simulink model "tinydl"  (R2025b)
settings: Solver=FixedStepAuto  StartTime=0.0  StopTime=inf  RelTol=1e-3  EnableMultiTasking=on
libraries: arduinolib x8
settings Model: ExtModeTrigDuration=2  Creator=Dogukan.kilinc  LastModifiedBy=Dogukan.kilinc
settings SolverCC: AutoInsertRateTranBlk=on
settings DataIOCC: ReturnWorkspaceOutputs=off
settings OptimizationCC: EnhancedBackFolding=on  PassReuseOutputArgsAs=Individual arguments  ZeroExternalMemoryAtStartup=off  ZeroInternalMemoryAtStartup=off  MaxStackSize=64  OptimizeBlockOrder=speed  DifferentSizesBufferReuse=on  OptimizationCustomize=off  EfficientTunableParamExpr=on
settings DebuggingCC: ParameterTunabilityLossMsg=error
settings HardwareCC: ProdBitPerPointer=32.0  ProdBitPerSizeT=32.0  ProdBitPerPtrDiffT=32.0  ProdLargestAtomicInteger=Long  ProdLargestAtomicFloat=Double  ProdWordSize=32.0  ProdHWDeviceType=ARM Compatible->ARM Cortex
settings SFSimCC: MATLABDynamicMemAlloc=off
settings RTWCC: SystemTargetFile=ert.tlc  HardwareBoard=Raspberry Pi Pico (Arduino Compatible)  TemplateMakefile=ert_default_tmf  Toolchain=Arduino ARM RP2040  BuildConfiguration=Faster Runs  Description=Embedded Coder
settings CodeAppCC: ForceParamTrailComments=on  IgnoreCustomStorageClasses=off  OperatorAnnotations=on  SimulinkDataObjDesc=on  SFDataObjDesc=on  InsertBlockDesc=on
settings ERTTargetCC: ExtModeTransport=3.0  ExtModeStaticAlloc=on  ExtModeAutomaticAllocSize=off  ExtModeStaticAllocSize=65536.0  ExtModeMexFile=ext_xcp  ExtModeIntrfLevel=Level2 - Open  InlinedParameterPlacement=Hierarchical  SupportContinuousTime=on  SupportVariableSizeSignals=on

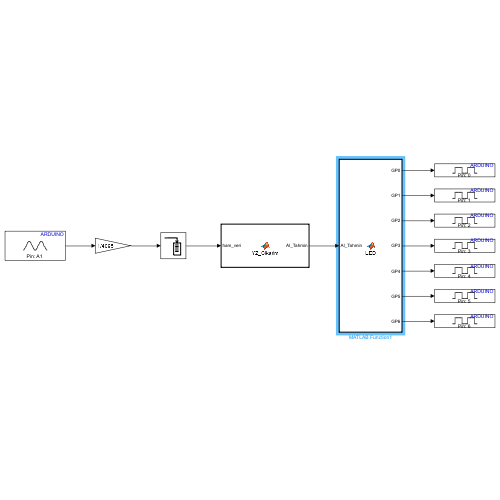
[thumbnail: Simulink's stored preview of the top-level diagram]
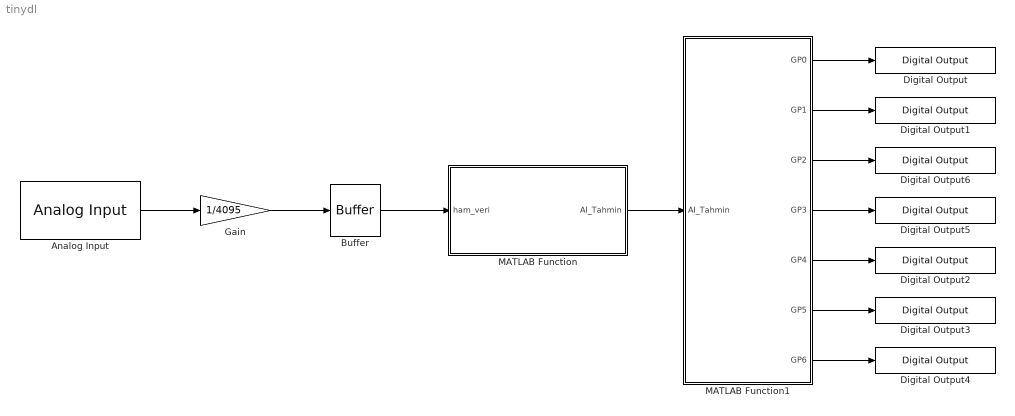
== system tinydl ==
  Analog Input : arduinolib/Analog Input  pinNumber=1  ReadResultsOnly=off  ConversionTriggerSource=Software  ExternalTriggerType=uint32( 0 )  OutputDataType=uint16  EnableConversionCompleteNotify=off  EnableOuputStatus=off  SampleTime=0.1  blockPlatform=arduino
  Buffer : Buffer  N=50  OutputFrames=off
  Digital Output : arduinolib/Digital Output  pinNumber=0  Direction=output  blockPlatform=arduino
  Digital Output1 : arduinolib/Digital Output  pinNumber=1  Direction=output  blockPlatform=arduino
  Digital Output2 : arduinolib/Digital Output  pinNumber=4  Direction=output  blockPlatform=arduino
  Digital Output3 : arduinolib/Digital Output  pinNumber=5  Direction=output  blockPlatform=arduino
  Digital Output4 : arduinolib/Digital Output  pinNumber=6  Direction=output  blockPlatform=arduino
  Digital Output5 : arduinolib/Digital Output  pinNumber=3  Direction=output  blockPlatform=arduino
  Digital Output6 : arduinolib/Digital Output  pinNumber=2  Direction=output  blockPlatform=arduino
  Gain : Gain  Gain=1/4095  OutDataTypeStr=double
  MATLAB Function : MATLAB Function  TreatAsAtomicUnit=on
  MATLAB Function1 : MATLAB Function  TreatAsAtomicUnit=on
  wires:
  Analog Input/1 -> Gain/1
  Gain/1 -> Buffer/1
  Buffer/1 -> MATLAB Function/1(ham_veri)
  MATLAB Function/1(AI_Tahmin) -> MATLAB Function1/1(AI_Tahmin)
  MATLAB Function1/1(GP0) -> Digital Output/1
  MATLAB Function1/2(GP1) -> Digital Output1/1
  MATLAB Function1/7(GP6) -> Digital Output4/1
  MATLAB Function1/6(GP5) -> Digital Output3/1
  MATLAB Function1/5(GP4) -> Digital Output2/1
  MATLAB Function1/3(GP2) -> Digital Output6/1
  MATLAB Function1/4(GP3) -> Digital Output5/1

== matlab function tinydl/MATLAB Function1 ==
  data: AI_Tahmin input; GP0 output; GP1 output; GP2 output; GP3 output; GP4 output; GP5 output; GP6 output
function [GP0, GP1, GP2, GP3, GP4, GP5, GP6] = LED(AI_Tahmin)
    % Hafızada tutulacak değişkenleri (sayacı) tanımlıyoruz
    persistent sayac
    persistent baslangic_bitti

    % Pico fişe İLK KEZ takıldığında değerleri sıfırla
    if isempty(sayac)
        sayac = 0;
        baslangic_bitti = false;
    end

    % --- HANGİ SAYININ GÖSTERİLECEĞİNE KARAR VER ---
    if ~baslangic_bitti
        % Eğer açılış animasyonu bitmediyse sayacı göster
        gosterilecek_deger = sayac;
        
        % Sayacı bir artır
        sayac = sayac + 1;
        
        % Eğer 9'a ulaştıysa başlangıç animasyonunu kalıcı olarak kapat
        if sayac > 9
            baslangic_bitti = true;
        end
    else
        % Açılış bittiyse artık sadece yapay zekanın (1 veya 2) sonucunu göster
        gosterilecek_deger = AI_Tahmin;
    end

    % --- 7-SEGMENT EKRAN YAKMA HARİTASI ---
    % Hangi rakam isteniyorsa onun LED'lerini (1) yak, diğerlerini (0) söndür
    switch gosterilecek_deger
        case 0
            GP0=1; GP1=1; GP2=1; GP3=1; GP4=1; GP5=1; GP6=0;
        case 1
            GP0=0; GP1=1; GP2=1; GP3=0; GP4=0; GP5=0; GP6=0;
        case 2
            GP0=1; GP1=1; GP2=0; GP3=1; GP4=1; GP5=0; GP6=1;
        case 3
            GP0=1; GP1=1; GP2=1; GP3=1; GP4=0; GP5=0; GP6=1;
        case 4
            GP0=0; GP1=1; GP2=1; GP3=0; GP4=0; GP5=1; GP6=1;
        case 5
            GP0=1; GP1=0; GP2=1; GP3=1; GP4=0; GP5=1; GP6=1;
        case 6
            GP0=1; GP1=0; GP2=1; GP3=1; GP4=1; GP5=1; GP6=1;
        case 7
            GP0=1; GP1=1; GP2=1; GP3=0; GP4=0; GP5=0; GP6=0;
        case 8
            GP0=1; GP1=1; GP2=1; GP3=1; GP4=1; GP5=1; GP6=1;
        case 9
            GP0=1; GP1=1; GP2=1; GP3=1; GP4=0; GP5=1; GP6=1;
        otherwise
            % Hata olursa tüm ekranı söndür
            GP0=0; GP1=0; GP2=0; GP3=0; GP4=0; GP5=0; GP6=0;
    end
end

== matlab function tinydl/MATLAB Function ==
  data: ham_veri input; AI_Tahmin output
function AI_Tahmin = YZ_Cikarim(ham_veri)
    %#codegen
    
    % 1. Yapay zeka modelimizi kalici (persistent) olarak gomuyoruz
    persistent net;
    if isempty(net)
        net = coder.loadDeepLearningNetwork('tiny_beyin.mat');
    end
    
    % 2. İŞTE YENİ SİHRİMİZ: Gelen veriyi ağa girmeden önce 'single' (32-bit) yapıyoruz!
    ham_veri_single = single(ham_veri);
    
    % 3. Veriyi dlarray'e (Time-Channel) ceviriyoruz
    dl_veri = dlarray(ham_veri_single, 'TC');
    
    % 4. Ağı çalıştırıp tahmin (olasılık) değerlerini alıyoruz
    olasiliklar = predict(net, dl_veri);
    
    % 5. dlarray formatından standart diziye çıkartıyoruz
    saf_olasilik = extractdata(olasiliklar);
    
    % 6. Hangi olasılık daha yüksekse onun indeksini (1: Kuru, 2: Nemli) buluyoruz
    [~, sinif_indeksi] = max(saf_olasilik);
    
    % 7. LCD bloğu 'double' beklediği için sonucu double olarak fırlatıyoruz
    AI_Tahmin = double(sinif_indeksi);
end
